simulink model "Block_Daigram_open_step_response"  (R2016a)
settings: Solver=ode45  StartTime=0.0  StopTime=50  RelTol=1e-3
settings Model: Creator=Muhammad Zubair  LastModifiedBy=Muhammad Zubair

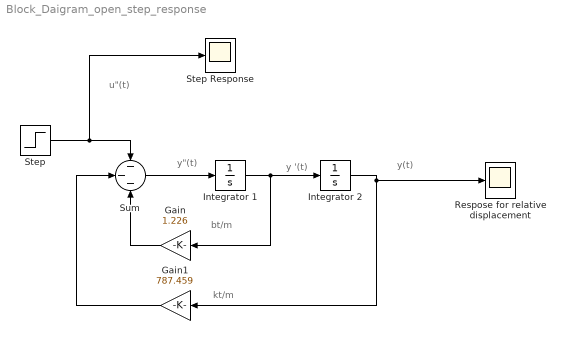
== system Block_Daigram_open_step_response ==
  note: u"(t)
  note: kt/m
  note: bt/m
  note: y(t)
  note: y '(t)
  note: y"(t)
  Gain : Gain  Gain=1.226
  Gain1 : Gain  Gain=787.459
  Integrator 1 : Integrator
  "Integrator 2 " : Integrator
  Respose for relative displacement : Scope
  Step : Step  Time=0.01  After=8  SampleTime=0
  Step Response : Scope
  Sum : Sum  Inputs=---
  wires:
  Sum/1 -> Integrator 1/1
  Integrator 1/1 -> Gain/1, "Integrator 2 "/1
  Gain/1 -> Sum/3
  Gain1/1 -> Sum/2
  "Integrator 2 "/1 -> Respose for relative displacement/1, Gain1/1
  Step/1 -> Sum/1, Step Response/1
